simulink model "FlightSimulation"  (R2025a)
settings: Solver=ode4  StartTime=0.0  StopTime=Inf  FixedStep=time.dt  MaxStep=0.001  RelTol=1e-3
values from neighbouring files (symbols this model uses):
  AeroModel = init_IREC2025_CFDModel()    [RunSimulink.m]
  const = setupConstants()    [RunSimulink.m]
  kfConsts = getKfConsts()    [RunSimulink.m]
  kfErrInds = getErrorKfInds()    [RunSimulink.m]
  kfInds = getKfInds()    [RunSimulink.m]
  kfParams = initNavParams(kins)    [RunSimulink.m]
  kins = HPRC_RocketKinematics()    [RunSimulink.m]
  launchLLA = [launchLat, launchLon, launchAlt]    [RunSimulink.m]
  MotorModel = initMotorModel()    [RunSimulink.m]
  w_ib_x = 1e-10    [RunSimulink.m]
  w_ib_y = 1e-10    [RunSimulink.m]
  w_ib_z = 1e-10    [RunSimulink.m]
undefined symbols (not defined in the file or in its folder): Earth, F, fractalcoef, Light, MIL, Receive, Send, Sim3dSensor, simCfg, time, WGS84, WMM2020
libraries: simulink x6, aerolibatmos2 x5, aerolibfltsims x2, sim3dlib x2, aerolibsim3d x2, mspsensorlib x1, aerolibnav x1, aerolibgravity2 x1, aerolib6dof2 x1, aerolibwind2 x1, simulink_extras x1, matrix_library x1
(part 2 of 2)

== matlab function FlightSimulation/Flight Computer/Navigator/Update Step/Mag Update/MATLAB Function ==
  data: navIn input Bus: kfParamsBus; navOut output Bus: kfParamsBus; kfInds parameter; kfErrInds parameter; kfConsts parameter; u_mag input
function navOut = magHeadingUpdate(navIn, kfInds, kfErrInds, kfConsts, u_mag)
    navOut = navIn;

    %% === Setup ===
    x_pred = navOut.x;
    P_min  = navOut.P;

    q  = x_pred(kfInds.quat);         % [w x y z]
    bm = x_pred(kfInds.magBias);      % Magnetometer bias

    %% === Measured field in body frame (bias corrected, normalized)
    m_b = u_mag(:) - bm;
    m_b = m_b / norm(m_b + 1e-8);  % normalize with epsilon to avoid NaNs

    %% === Rotate to NED and project to horizontal plane
    R_BN = quat2rotm(q');             % Body-to-NED
    m_n = R_BN * m_b;
    m_n(3) = 0;

    if norm(m_n) < 1e-3
        return;  % Insufficient horizontal component to resolve heading
    end

    m_n = m_n / norm(m_n);
    yaw_meas = atan2(-m_n(2), m_n(1));  % Heading in NED frame (E/N)

    %% === Predicted yaw from current quaternion
    qw = q(1); qx = q(2); qy = q(3); qz = q(4);
    yaw_pred = atan2(2*(qw*qz + qx*qy), 1 - 2*(qy^2 + qz^2));

    %% === Innovation ===
    y = wrapToPi(yaw_meas - yaw_pred);

    %% === Jacobian: ∂yaw/∂(δθ)
    dq = 1e-5;
    H_theta = zeros(1, 3);
    for i = 1:3
        dtheta = zeros(3,1);
        dtheta(i) = dq;
        dq_pert = smallAngleQuaternion(dtheta);
        q_pert = quatmultiply(dq_pert', q')';
        R_pert = quat2rotm(q_pert');
        m_n_pert = R_pert * m_b;
        m_n_pert(3) = 0;
        if norm(m_n_pert) < 1e-3
            return;
        end
        m_n_pert = m_n_pert / norm(m_n_pert);
        yaw_pert = atan2(-m_n_pert(2), m_n_pert(1));
        H_theta(i) = (yaw_pert - yaw_pred) / dq;
    end

    %% === Jacobian: ∂yaw/∂(bm)
    H_bm = zeros(1, 3);
    for i = 1:3
        db = zeros(3,1);
        db(i) = dq;
        m_b_pert = (u_mag(:) - bm - db);  % Subtract db for ∂h/∂bm = -∂h/∂m_b
        m_b_pert = m_b_pert / norm(m_b_pert + 1e-8);
        m_n_pert = R_BN * m_b_pert;
        m_n_pert(3) = 0;
        if norm(m_n_pert) < 1e-3
            return;
        end
        m_n_pert = m_n_pert / norm(m_n_pert);
        yaw_pert = atan2(-m_n_pert(2), m_n_pert(1));
        H_bm(i) = (yaw_pert - yaw_pred) / dq;
    end

    %% === Assemble Kalman update ===
    H = zeros(1, kfErrInds.maxStateIndex);
    H(1, kfErrInds.theta) = H_theta;
    H(1, kfErrInds.magBias) = H_bm;

    R = deg2rad(3)^2;  % 3 deg stddev → variance

    S = H * P_min * H' + R;
    K = P_min * H' / S;
    dx = K * y;

    %% === Apply correction to nominal state ===
    delta_q = smallAngleQuaternion(dx(kfErrInds.theta));
    q_update = quatmultiply(delta_q', q')';
    q_update = q_update / norm(q_update);

    x_update = x_pred;
    x_update(kfInds.quat)     = q_update;
    x_update(kfInds.magBias)  = x_update(kfInds.magBias) + dx(kfErrInds.magBias);

    navOut.x = x_update;

    %% === Covariance Update (Joseph Form) ===
    I = eye(size(P_min));
    navOut.P = (I - K * H) * P_min * (I - K * H)' + K * R * K';
    navOut.P = 0.5 * (navOut.P + navOut.P');  % Force symmetry
end

== matlab function FlightSimulation/Flight Computer/Sensor Bus/MATLAB Function2 ==
  data: h input; P_true output; const parameter; P_corr output
function [P_true, P_corr] = corruptBarometer(h, const)

rng(42);

LPS22_PARAMS = getLPS22HHParams();

P_true = const.P0 * (1 - (const.L * h) / const.T0)^(const.g_e*const.M / (const.R*const.L));

bias = LPS22_PARAMS.bias;
sf   = LPS22_PARAMS.sf;
k2   = LPS22_PARAMS.k2;
k3   = LPS22_PARAMS.k3;

noise = LPS22_PARAMS.noise * randn();

P_corr = P_true + bias + noise;

== matlab function FlightSimulation/Flight Computer/Navigator/Update Step/Baro Update/MATLAB Function ==
  data: navIn input Bus: kfParamsBus; navOut output Bus: kfParamsBus; kfInds parameter; kfConsts parameter; u_baro input; const parameter
function navOut = magHeadingUpdate(navIn, kfInds, kfConsts, u_baro, const)
    navOut = navIn;

    if any(isnan(navOut.x_pred))
        navOut.x = navOut.x_pred;
        navOut.P = navOut.P_min;
        return;
    end

    %% === Setup ===
    x_pred = navOut.x;
    P_min  = navOut.P;

    % Convert Pressure to Altitude
    h_baro = (const.T0 / const.L) * (1 - (u_baro / const.P0)^(const.R * const.L / const.g_e));

    z_pred = x_pred(kfInds.pos(3));
    h_pred = -h_baro;

    % Innovation
    y = h_baro - h_pred;

    %% Measurement Jacobian
    H = zeros(1, length(x_pred));
    H(kfInds.pos(3)) = -1;

    % Measurement Noise
    R_baro = (0.3)^2; % [m]

    % Kalman Gain and Update
    S = H * P_min * H' + R_baro;
    K = P_min * H' / S;

    x_update = x_pred + K * y;
    navOut.x = x_update;

    P_update = (eye(length(x_pred)) - K * H) * P_min;
    navOut.P = 0.5 * (P_update + P_update');
    

end

== matlab function FlightSimulation/Flight Computer/Sensor Bus/ICM20948/MATLAB Function 2 ==
  data: gyro_true input; gyro_corr output
function gyro_corr = corruptSensorReading(gyro_true)

ICM20948_PARAMS = getICM20948Params();


gyro_corr = applySensorModel(gyro_true, ICM20948_PARAMS.gyro);

== matlab function FlightSimulation/Flight Computer/Navigator/Initialize Nav/Initialize State/MATLAB Function2 ==
  data: a_b input; q_0 output; m_b input
function q_0 = computeInitialQuaternion_(a_b, m_b)

    if(~(norm(a_b) > 2))
        q_0 = [NaN; NaN; NaN; NaN];
        return;
    end


    q_0 = computeInitialQuaternion(a_b, m_b);

== matlab function FlightSimulation/Flight Computer/Navigator/Initialize Nav/Initialize State/MATLAB Function3 ==
  data: initFlagLoop input; q_0 input; x_0 output; kfInds parameter; kfParams parameter; initFlag output
function [x_0, initFlag]= initializeState_(initFlagLoop, q_0, kfInds, kfParams)
%#codegen

    x_0 = kfParams.x;

    if(initFlagLoop == 1)
        initFlag = 1;
        return;
    end

    if any(isnan(q_0))
        initFlag = 0;
    
    else 
        x_0(kfInds.quat) = q_0;

        x_0(kfInds.g)
        initFlag = 1;
    end

== matlab function FlightSimulation/Flight Computer/Navigator/MATLAB Function ==
  data: navIn input Bus: kfParamsBus; navOut output Bus: kfParamsBus; kfInds parameter; kfErrInds parameter; kfConsts parameter; sf_b input; w_ib_b input; sf_b_prev input; w_ib_b_prev input; time parameter
function navOut = navPred(navIn, kfInds, kfErrInds, kfConsts, sf_b, w_ib_b, sf_b_prev, w_ib_b_prev, time)

u_k = [w_ib_b(:); sf_b(:)];

u_k1 = [w_ib_b_prev(:); sf_b_prev(:)];

navOut = navIn;

[navOut.x_pred, navOut.f_pred] = propABAM2(navIn.x, navIn.f_pred, u_k, u_k1, kfInds, time);

phi = predictionJacobian(navIn.x, u_k, kfInds, kfErrInds, kfConsts, time);

navOut.P_min = phi * navOut.P * phi' + navOut.Q_k;

== matlab function FlightSimulation/Flight Computer/Navigator/Update Step/Gravity Update/MATLAB Function ==
  data: navIn input Bus: kfParamsBus; navOut output Bus: kfParamsBus; kfInds parameter; kfErrInds parameter; kfConsts parameter; accelMeas input
function navOut = gravityUpdate(navIn, kfInds, kfErrInds, kfConsts, accelMeas)
% GRAVITYUPDATE - Kalman update using accelerometer to estimate gravity magnitude
% INPUTS:
%   navIn     - Input navigation state structure (with x_pred, P_min)
%   kfInds    - State indices structure (fields: quat, accelBias, g, etc.)
%   kfErrInds - Error state indices structure (fields: theta, accelBias, g, etc.)
%   kfConsts  - Filter constants (including R_grav)
%   accelMeas - [3x1] Accelerometer measurement (in body frame)
% OUTPUT:
%   navOut    - Updated navigation state structure (with x, P)

    navOut = navIn;

    % Skip update if prediction is invalid
    if any(isnan(navOut.x_pred))
        navOut.x = navOut.x_pred;
        navOut.P = navOut.P_min;
        return;
    end

    %% === Setup ===
    x_pred = navOut.x_pred;
    P_min  = navOut.P_min;

    q  = x_pred(kfInds.quat);        % Quaternion: body-to-NED
    ba = x_pred(kfInds.accelBias);   % Accel bias
    g  = x_pred(kfInds.g);           % Estimated gravity magnitude (scalar)

    G_NED = [0; 0; g];              % Gravity vector in NED
    R_NB = quat2rotm(q');            % Rotation body-to-NED

    %% === Measurement Prediction ===
    accel_pred = R_NB' * G_NED;     % Predicted accel in body frame
    accel_meas = accelMeas(:) - ba;          % Measured accel in body frame

    % Optional: Skip update if under high dynamics
    if abs(norm(accel_meas) - g) > 1.0
        return;
    end

    y = accel_meas - accel_pred;        % Residual

    %% === Measurement Jacobian ===
    H = zeros(3, kfErrInds.maxStateIndex);

    % Sensitivity to attitude error (δθ)
    H(:, kfErrInds.theta) = -R_NB * skew(G_NED);

    % Sensitivity to accel bias
    H(:, kfErrInds.accelBias) = -eye(3);

    % Sensitivity to gravity magnitude
    H(:, kfErrInds.g) = [0; 0; -1];

    %% === Measurement Noise
    R = kfConsts.R_grav;

    %% === Kalman Gain
    S = H * P_min * H' + R;
    K = P_min * H' / S;
    dx = K * y;

    %% === Apply Correction ===
    delta_theta = dx(kfErrInds.theta);
    angle = norm(delta_theta);

    % Limit correction angle to 10 deg
    if angle > deg2rad(10)
        delta_theta = delta_theta * (deg2rad(10) / angle);
    end

    delta_q = smallAngleQuaternion(delta_theta);
    q_update = quatmultiply(delta_q', q')';

    x_update = x_pred;
    x_update(kfInds.quat)       = q_update / norm(q_update);  % Normalize quaternion
    x_update(kfInds.accelBias)  = x_update(kfInds.accelBias) + dx(kfErrInds.accelBias);
    x_update(kfInds.g)          = x_update(kfInds.g) + dx(kfErrInds.g);  % <-- gravity update added

    %% === Covariance Update ===
    I = eye(size(P_min));
    P_update = (I - K * H) * P_min * (I - K * H)' + K * R * K';

    %% === Save to Output
    navOut.x = x_update;
    navOut.P = 0.5 * (P_update + P_update');  % Force symmetry

end

== matlab function FlightSimulation/Flight Computer/Navigator/Update Step/MATLAB Function ==
  data: navIn input Bus: kfParamsBus; navOut output Bus: kfParamsBus; kfInds parameter; kfConsts parameter; time parameter
function navOut = passiveUpdate(navIn, kfInds, kfConsts, time)

navOut = navIn;

navOut.x = navOut.x_pred;
navOut.P = navOut.P_min;

navOut.P = (navOut.P + navOut.P') * 0.5;

== matlab function FlightSimulation/Unreal/MATLAB Function ==
  data: P_E input; P_T output; refLLA input
function P_T = ecef2ned_pos_(P_E, refLLA)

P_T = ecef2ned_pos(P_E, refLLA);

== stateflow chart FlightSimulation/Flight Computer/State Machine/Chart ==
  state PreLaunch
  state Launch
    entry:
    state=1
    guid=0
  state Burnout
    entry:
    state=2
    guid=0
  state Guidance
    entry:
    state=3
    guid=1
  state Apogee
    entry:
    state=4
    guid=0
  (default) -> PreLaunch : {state=0}
  PreLaunch -> Launch : [A_b_x > 3]
  Launch -> Burnout : [A_b_x < 1]
  Burnout -> Guidance : [after(1, sec)]
  Guidance -> Apogee : [v_vert < 1]
  data: A_b_x input; v_vert input; guid output; state output

== matlab function FlightSimulation/Flight Computer/Sensor Bus/MATLAB Function ==
  data: u input; R_BT output
function R_BT = nedToBody_(u)

R_BT = eul_NED2BODY(u);

== matlab function FlightSimulation/Flight Computer/Sensor Bus/ICM20948/MATLAB Function ==
  data: a_b input; sf_true output; R_BT input
function sf_true = accel2sf_(a_b, R_BT)

sf_true = accel2sf(a_b, R_BT);

== matlab function FlightSimulation/Flight Computer/Sensor Bus/ICM20948/MATLAB Function 1 ==
  data: sf_true input; sf_corr output
function sf_corr = corruptSensorReading(sf_true)

ICM20948_PARAMS = getICM20948Params();


sf_corr = applySensorModel(sf_true, ICM20948_PARAMS.accel);

== matlab function FlightSimulation/Flight Computer/Sensor Bus/MATLAB Function1 ==
  data: B_true input; B_corr output
function B_corr = corruptSensorReading(B_true)

MMC5983_PARAMS = getMMC5983Params();

B_corr = applySensorModel(B_true, MMC5983_PARAMS);

== matlab function FlightSimulation/Flight Computer/Navigator/Update Step/GPS Update/MATLAB Function ==
  data: navIn input Bus: kfParamsBus; navOut output Bus: kfParamsBus; kfInds parameter; kfErrInds parameter; kfConsts parameter; u_k input; time parameter
function navOut = gpsUpdate(navIn, kfInds, kfErrInds, kfConsts, u_k, time)

    % Force column
    u_k = u_k(:);
    navOut = navIn;

    %% === Setup ===
    x_pred = navOut.x;
    P_min  = navOut.P;

    % Measurement model: position only
    z = u_k(1:3);                  % GPS position measurement
    h = x_pred(kfInds.pos);        % Predicted position
    y = z - h;                     % Innovation

    %% === Measurement Jacobian wrt error state ===
    H = zeros(3, kfErrInds.maxStateIndex);
    H(:, kfErrInds.pos) = eye(3);  % Only sensitive to position errors

    %% === Kalman Update ===
    R = kfConsts.R_gps;  % Should be 3x3 covariance of GPS measurement
    S = H * P_min * H' + R;
    K = P_min * H' / S;

    dx = K * y;  % Error state correction

    %% === Apply Correction to Nominal State ===
    x_update = x_pred;

    % Apply additive position correction
    x_update(kfInds.pos) = x_update(kfInds.pos) + dx(kfErrInds.pos);

    % Optional: could add velocity or clock bias terms here if needed

    % Apply corrected state
    navOut.x = x_update;

    % Joseph form update (for stability)
    I = eye(size(P_min));
    navOut.P = I - K * H;
    navOut.P = navOut.P * P_min * navOut.P' + K * R * K';
    navOut.P = 0.5 * (navOut.P + navOut.P');  % Enforce symmetry

end

== matlab function FlightSimulation/Flight Dynamics/MATLAB Function ==
  data: P_E input; P_T output; refLLA input
function P_T = ecef2ned_pos_(P_E, refLLA)

P_T = ecef2ned_pos(P_E, refLLA);
